simulink model "DCMotorSpeedControl"  (R2015b)
settings: Solver=VariableStepAuto  StartTime=0.0  StopTime=0.02  RelTol=1e-3
libraries: LocalLib x2
settings Model: Creator=jje  LastModifiedBy=jje

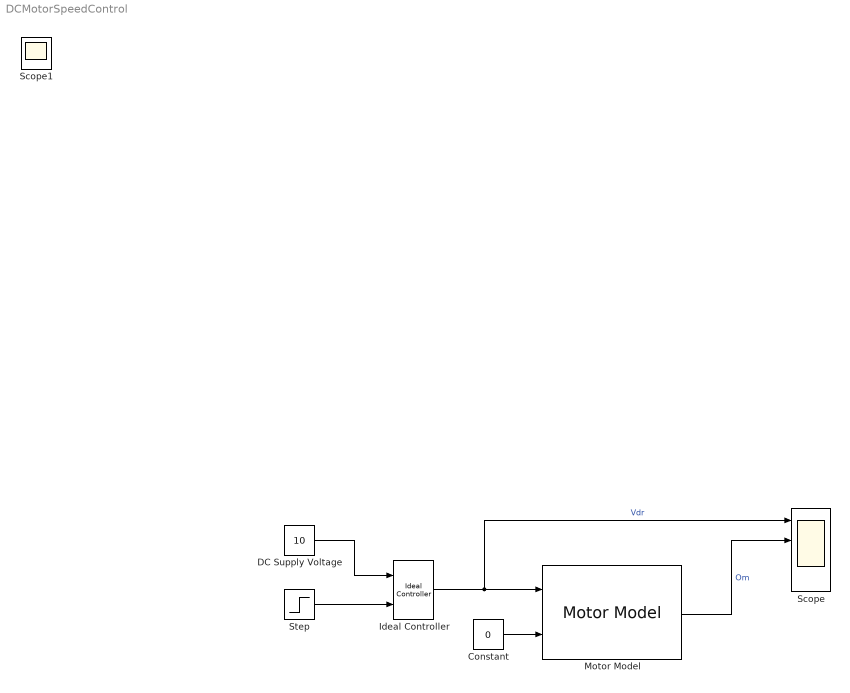
== system DCMotorSpeedControl ==
  Constant : Constant  Value=0
  DC Supply Voltage : Constant  Value=10
  Ideal Controller : LocalLib/Ideal Controller
  Motor Model : LocalLib/Motor Model
  Scope : Scope  NumInputPorts=4
  Step : Step  Time=0.01  SampleTime=0
  Scope1 : Scope
  wires:
  DC Supply Voltage/1 -> Ideal Controller/1
  Ideal Controller/1 -> Motor Model/1, Scope/1  "Vdr"
  Constant/1 -> Motor Model/2
  Step/1 -> Ideal Controller/2
  Motor Model/1 -> Scope/2  "Om"
